simulink model "Ball_Detection"  (R2020a)
settings: Solver=VariableStepAuto  StartTime=0.0  StopTime=inf  RelTol=1e-3
undefined symbols (not defined in the file or in its folder): none, serial, videoinput
libraries: instrumentlib x2, visiontextngfix x1, imaqlib x1, visionsinks x1
settings Model: Creator=vince  LastModifiedBy=vince

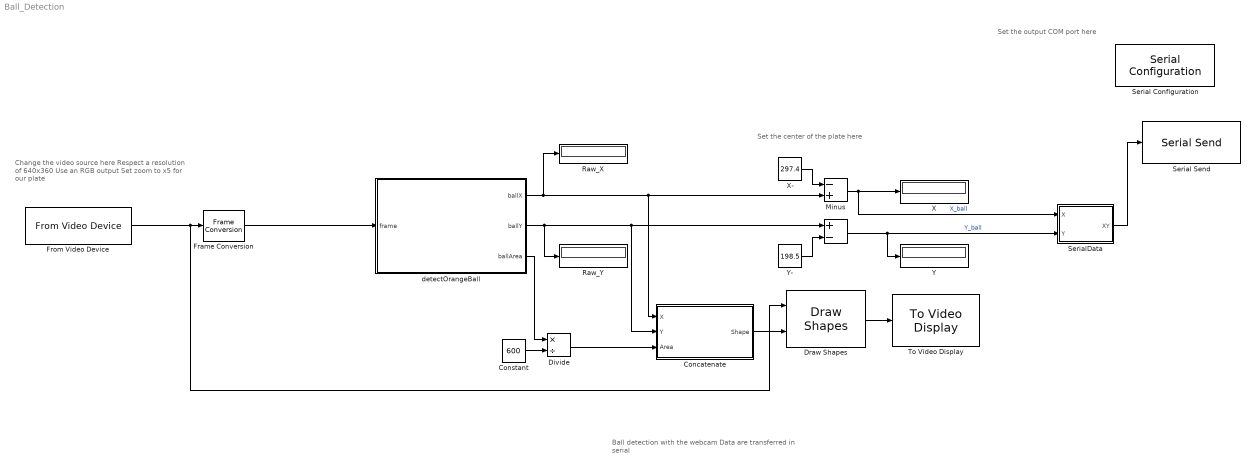
== system Ball_Detection ==
  note: Set the center of the plate here
  note: Set the output COM port here
  note: Change the video source here
      | Respect a resolution of 640x360
      | Use an RGB output
      | Set zoom to x5 for our plate
  note: Ball detection with the webcam
      | Data are transferred in serial
  " " : Sum  Inputs=+-
  Concatenate : MATLAB Function  TreatAsAtomicUnit=on
  Constant : Constant  Value=600
  Divide : Product  Inputs=*/
  Draw Shapes : visiontextngfix/Draw Shapes  shape=Circles  fill=on  lineWidth=1  fillClrSource=Specify via dialog  display=User-specified value  intensity=200  color=[255 255 000]  opacity=0.6  viewport=Entire image  antialiasing=off  inType=Obsolete  imagePorts=One multidimensional signal  roundingMode=Floor  overflowMode=off  memoryMode=Specify word length  memoryWordLength=16  prodOutputMode=Binary point scaling  prodOutputWordLength=32  prodOutputFracLength=14  memoryFracLength=15
  Frame Conversion : FrameConversion  OutFrame=Sample-based
  From Video Device : imaqlib/From Video Device  DeviceMenu=winvideo 1 (Integrated Camera)  Device=winvideo 1 (Integrated Camera)  ObjConstructor=videoinput('winvideo', 1)  VideoFormatMenu=YUY2_640x360  VideoFormat=YUY2_640x360  VideoSource=input1  ROIPosition=[0 0 360 640]  EnableHWTrigger=off  TriggerConfiguration=none/none  SampleTime=1/30  OutputPortsMode=One multidimensional signal  DataType=single  CanDoHWTrigger=no  ReturnedColorSpace=rgb  BlockHandle=32.0001  ROIWidth=640  ROIHeight=360  ROIColumn=0  ROIRow=0  EngXMLPath=C:\Program Files\MATLAB\R2020a\toolbox\imaq\imaq\private  DevXMLPath=C:\ProgramData\MATLAB\SupportPackages\R2020a\toolbox\imaq\supportpackages\genericvideo\adaptor\win64  EngLibPath=C:\Program Files\MATLAB\R2020a\toolbox\imaq\imaqblks\imaqmex\win64  ColorSpace=rgb  BayerSensorAlignment=grbg  ImaqMode=off
  Minus : Sum  Inputs=-+
  Raw_X : Display
  Raw_Y : Display
  Serial Configuration : instrumentlib/Serial Configuration  Priority=-200000  ComPortMenu=<Please select a port...>  ComPort=COM7  ObjConstructor=serial('COM7');  BaudRate=9600  DataBits=8  Parity=none  StopBits=1  FlowControl=none  Timeout=10  ByteOrder=LittleEndian
  Serial Send : instrumentlib/Serial Send  ComPortMenu=<Please select a port...>  ComPort=COM7  ObjConstructor=serial('COM7');  Terminator=<none>  EnableBlockingMode=on
  SerialData : MATLAB Function  TreatAsAtomicUnit=on
  To Video Display : visionsinks/To Video Display  windowSizeMode=Normal  openAtMdlStart=on  fullScreen=off  videoWindowX=456  videoWindowY=181  saveWindowSize=off  videoWindowWidth=1325  videoWindowHeight=766  inputColorFormat=RGB  inputType=Obsolete  imagePorts=One multidimensional signal  OutputDevice=On-screen video monitor  dataOrg=Column-major  isWindowOpen=off
  X : Display
  X- : Constant  Value=297.4
  Y : Display
  Y- : Constant  Value=198.5
  detectOrangeBall : MATLAB Function  TreatAsAtomicUnit=on  RTWFcnName=detectOrangeBall
  wires:
  Frame Conversion/1 -> detectOrangeBall/1(frame)
  From Video Device/1 -> Draw Shapes/1, Frame Conversion/1
  detectOrangeBall/1(ballX) -> Minus/2, Concatenate/1(X), Raw_X/1
  detectOrangeBall/3(ballArea) -> Divide/1
  Draw Shapes/1 -> To Video Display/1
  detectOrangeBall/2(ballY) -> " "/1, Concatenate/2(Y), Raw_Y/1
  Concatenate/1(Shape) -> Draw Shapes/2
  Constant/1 -> Divide/2
  Divide/1 -> Concatenate/3(Area)
  X-/1 -> Minus/1
  Y-/1 -> " "/2
  Minus/1 -> SerialData/1(X), X/1  "X_ball"
  " "/1 -> Y/1, SerialData/2(Y)  "Y_ball"
  SerialData/1(XY) -> Serial Send/1

== matlab function Ball_Detection/Concatenate ==
  data: X input size=[2]; Shape output size=[1 3]; Y input size=[2]; Area input size=[2]
function Shape = Concatenate(X,Y ,Area)
Shape=[int32(X(1)), int32(Y(1)), int32(Area(1))];

== matlab function Ball_Detection/detectOrangeBall ==
  data: ballX output size=[2]; ballY output size=[2]; frame input; ballArea output size=[2]
function [ballX, ballY, ballArea] = detectOrangeBall(frame)
% Create the default minimum and maximum HSV values for orange color
orangeMin = [0.05 0.4 0.5];
orangeMax = [0.15 1.0 1.0];
ballArea = int32(0); % Fixed size for Simulink
DefaultX= int32(297.4);
DefaultY= int32(198.5);
% Create a blob analysis object
blobAnalyzer = vision.BlobAnalysis('MinimumBlobArea', 100, 'MaximumBlobArea', 10000);

while true
    % Check if the input frame is empty
    if isempty(frame)
        ballX = DefaultX;
        ballY = DefaultY;
        ballArea = int32(0);
        break;
    end
    
    % Convert the frame to HSV color space
    hsv = rgb2hsv(frame);
    
    % Create a mask for the orange color
    mask = (hsv(:,:,1) >= orangeMin(1)) & (hsv(:,:,1) <= orangeMax(1)) & ...
           (hsv(:,:,2) >= orangeMin(2)) & (hsv(:,:,2) <= orangeMax(2)) & ...
           (hsv(:,:,3) >= orangeMin(3)) & (hsv(:,:,3) <= orangeMax(3));
       
    % Perform blob analysis on the mask
    [areas, centroids] = step(blobAnalyzer, mask);
    
    % Find the largest blob in the image
    index = [];
    if ~isempty(areas)
        [~, index] = max(areas);
        ballX = int32(centroids(index, 1));
        ballY = int32(centroids(index, 2));
        ballArea = areas(index);
    else
        ballX = DefaultX;
        ballY = DefaultY;
        ballArea = int32(0)
        break; % No ball has been found
    end
    
    % Output the centroid and area of the largest blob
    if ~isempty(centroids)
        ballX = int32(centroids(index, 1));
        ballY = int32(centroids(index, 2));
        ballArea = areas(index);
        break;
    end
end

== matlab function Ball_Detection/SerialData ==
  data: X input size=[2]; XY output size=[1 2]; Y input size=[2]
function XY = SerialData(X , Y)
    x = int32(X(:)); % Convert X to a column vector and cast to int32
    y = int32(Y(:)); % Convert Y to a column vector and cast to int32
    XY = [x(1), y(1)]; % Take the first element of X and Y and concatenate into a 1-by-2 matrix
end
